simulink model "modlQuadcopter"  (R2024a)
settings: Solver=FixedStepAuto  StartTime=0.0  StopTime=CNFG_TEND  FixedStep=CNFG_TSTEP  RelTol=1e-3
undefined symbols (not defined in the file): BATT, CNST, DiscIntNeverNeededParam, MOTR, PROP, QUAD
libraries: vrlib x1, matrix_library x1
settings Model: Creator=anant  LastModifiedBy=anant

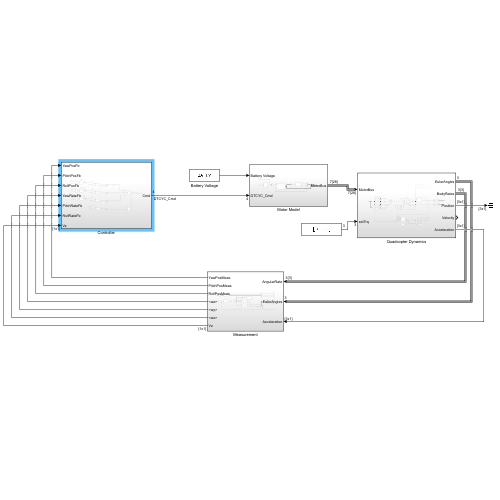
[thumbnail: Simulink's stored preview of the top-level diagram]
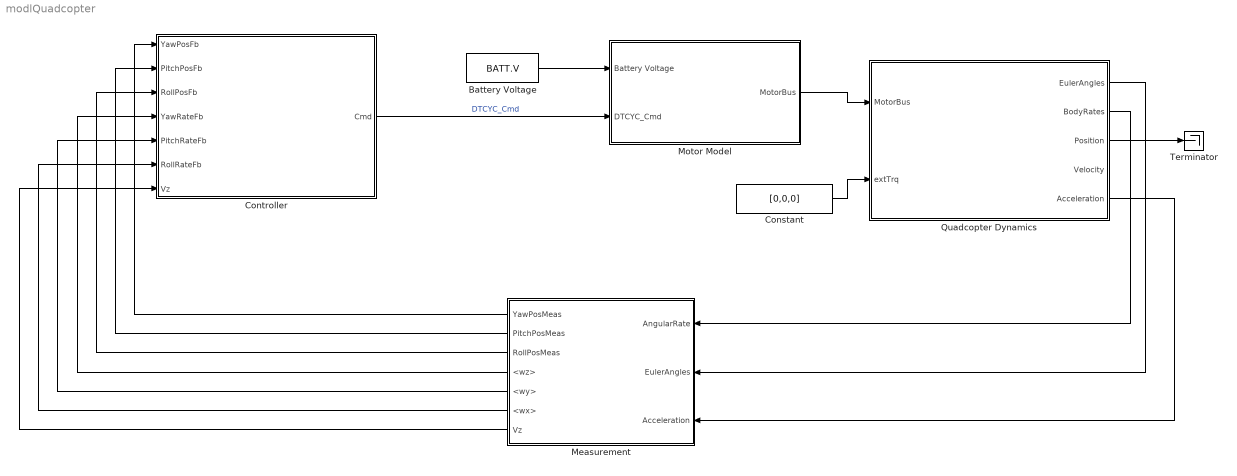
== system modlQuadcopter ==
  Battery Voltage : Constant  Value=BATT.V  SampleTime=0
  Constant : Constant  Value=[0,0,0]
  Controller : Subsystem
  Measurement : Subsystem
  Motor Model : Subsystem
  Quadcopter Dynamics : Subsystem
  Terminator : Terminator
  wires:
  Battery Voltage/1 -> Motor Model/1(Battery Voltage)
  Controller/1(Cmd) -> Motor Model/2(DTCYC_Cmd)  "DTCYC_Cmd"
  Motor Model/1(MotorBus) -> Quadcopter Dynamics/1(MotorBus)
  Quadcopter Dynamics/1(EulerAngles) -> Measurement/2(EulerAngles)
  Constant/1 -> Quadcopter Dynamics/2(extTrq)
  Quadcopter Dynamics/5(Acceleration) -> Measurement/3(Acceleration)
  Quadcopter Dynamics/2(BodyRates) -> Measurement/1(AngularRate)
  Measurement/1(YawPosMeas) -> Controller/1(YawPosFb)
  Measurement/2(PitchPosMeas) -> Controller/2(PitchPosFb)
  Measurement/3(RollPosMeas) -> Controller/3(RollPosFb)
  Measurement/4(<wz>) -> Controller/4(YawRateFb)
  Measurement/5(<wy>) -> Controller/5(PitchRateFb)
  Measurement/6(<wx>) -> Controller/6(RollRateFb)
  Measurement/7(Vz) -> Controller/7(Vz)
  Quadcopter Dynamics/3(Position) -> Terminator/1

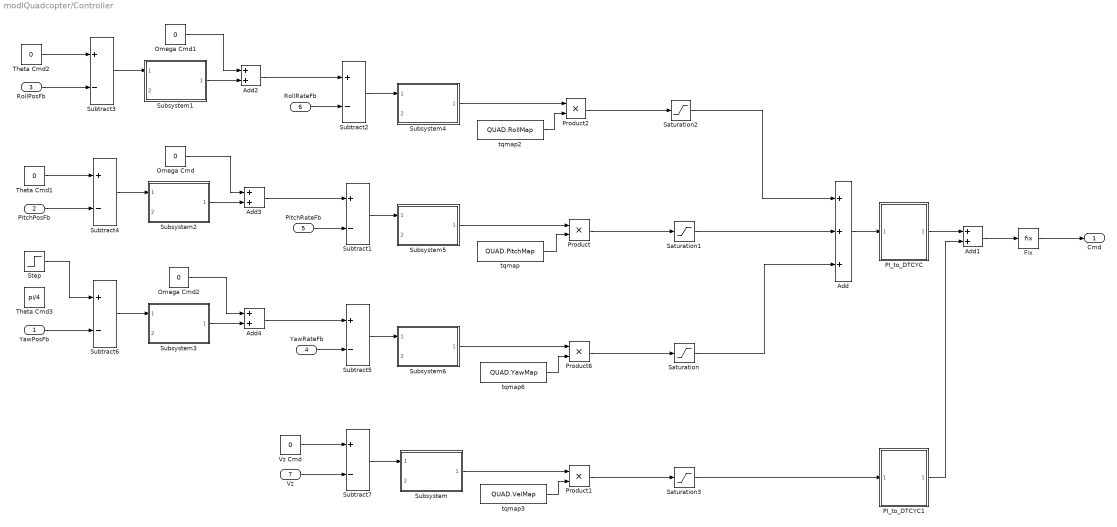
== system modlQuadcopter/Controller ==
  YawPosFb : Inport
  PitchPosFb : Inport  Port=2
  RollPosFb : Inport  Port=3
  YawRateFb : Inport  Port=4
  PitchRateFb : Inport  Port=5
  RollRateFb : Inport  Port=6
  Vz : Inport  Port=7
  Add : Sum  Inputs=+++
  Add{1..4} (4 alike) : Sum
  Fix : Rounding  Operator=fix
  Omega Cmd : Constant  Value=0
  Omega Cmd1 : Constant  Value=0
  Omega Cmd2 : Constant  Value=0
  PI_to_DTCYC : Subsystem  ReferencedSubsystem=subrMap  XL=-1  XU=1  YL=0  YU=500
  PI_to_DTCYC1 : Subsystem  ReferencedSubsystem=subrMap  XL=-1  XU=1  YL=1000  YU=2000
  Product{,1..2,6} (4 alike) : Product
  Saturation : Saturate  UpperLimit=0.2  LowerLimit=-0.2
  Saturation1 : Saturate  UpperLimit=0.4  LowerLimit=-0.4
  Saturation2 : Saturate  UpperLimit=0.4  LowerLimit=-0.4
  Saturation3 : Saturate  UpperLimit=1  LowerLimit=-1
  Step : Step  Time=0  After=0  SampleTime=0
  Subsystem : Subsystem  ReferencedSubsystem=subrPID  Kp=0.7  Ki=0.07  Kd=0  Ki_Sat=inf  TSTEP=CNTR.TSTEP
  Subsystem1 : Subsystem  ReferencedSubsystem=subrPID  Kp=20  Ki=0  Kd=0  Ki_Sat=inf  TSTEP=CNTR.TSTEP
  Subsystem2 : Subsystem  ReferencedSubsystem=subrPID  Kp=30  Ki=0  Kd=0  Ki_Sat=inf  TSTEP=CNTR.TSTEP
  Subsystem3 : Subsystem  ReferencedSubsystem=subrPID  Kp=5  Ki=0  Kd=0  Ki_Sat=inf  TSTEP=CNTR.TSTEP
  Subsystem4 : Subsystem  ReferencedSubsystem=subrPID  Kp=0.2  Ki=0  Kd=0  Ki_Sat=inf  TSTEP=CNTR.TSTEP
  Subsystem5 : Subsystem  ReferencedSubsystem=subrPID  Kp=0.2  Ki=0  Kd=0  Ki_Sat=inf  TSTEP=CNTR.TSTEP
  Subsystem6 : Subsystem  ReferencedSubsystem=subrPID  Kp=0.2  Ki=0  Kd=0  Ki_Sat=inf  TSTEP=CNTR.TSTEP
  Subtract{1..7} (7 alike) : Sum  Inputs=+-
  Theta Cmd1 : Constant  Value=0
  Theta Cmd2 : Constant  Value=0
  Theta Cmd3 : Constant  Value=pi/4
  Vz Cmd : Constant  Value=0
  tqmap : Constant  Value=QUAD.PitchMap
  tqmap2 : Constant  Value=QUAD.RollMap
  tqmap3 : Constant  Value=QUAD.VelMap
  tqmap6 : Constant  Value=QUAD.YawMap
  Cmd : Outport
  wires:
  Product6/1 -> Saturation/1
  Add2/1 -> Subtract2/1
  RollPosFb/1 -> Subtract3/2
  tqmap2/1 -> Product2/2
  tqmap6/1 -> Product6/2
  tqmap/1 -> Product/2
  RollRateFb/1 -> Subtract2/2
  Subtract2/1 -> Subsystem4/1
  Product/1 -> Saturation1/1
  PI_to_DTCYC/1 -> Add1/1
  Subtract1/1 -> Subsystem5/1
  Fix/1 -> Cmd/1
  PitchRateFb/1 -> Subtract1/2
  YawRateFb/1 -> Subtract5/2
  Product2/1 -> Saturation2/1
  Add/1 -> PI_to_DTCYC/1
  PI_to_DTCYC1/1 -> Add1/2
  Add1/1 -> Fix/1
  Add4/1 -> Subtract5/1
  Vz Cmd/1 -> Subtract7/1
  Vz/1 -> Subtract7/2
  Subtract7/1 -> Subsystem/1
  Subsystem/1 -> Product1/1
  tqmap3/1 -> Product1/2
  Product1/1 -> Saturation3/1
  Saturation3/1 -> PI_to_DTCYC1/1
  Subtract3/1 -> Subsystem1/1
  Omega Cmd1/1 -> Add2/1
  Theta Cmd2/1 -> Subtract3/1
  Subsystem1/1 -> Add2/2
  Omega Cmd/1 -> Add3/1
  Subsystem2/1 -> Add3/2
  Subtract4/1 -> Subsystem2/1
  PitchPosFb/1 -> Subtract4/2
  Theta Cmd1/1 -> Subtract4/1
  Add3/1 -> Subtract1/1
  Subsystem3/1 -> Add4/2
  YawPosFb/1 -> Subtract6/2
  Step/1 -> Subtract6/1
  Subsystem5/1 -> Product/1
  Subsystem6/1 -> Product6/1
  Subsystem4/1 -> Product2/1
  Omega Cmd2/1 -> Add4/1
  Saturation2/1 -> Add/1
  Saturation1/1 -> Add/2
  Saturation/1 -> Add/3
  Subtract5/1 -> Subsystem6/1
  Subtract6/1 -> Subsystem3/1

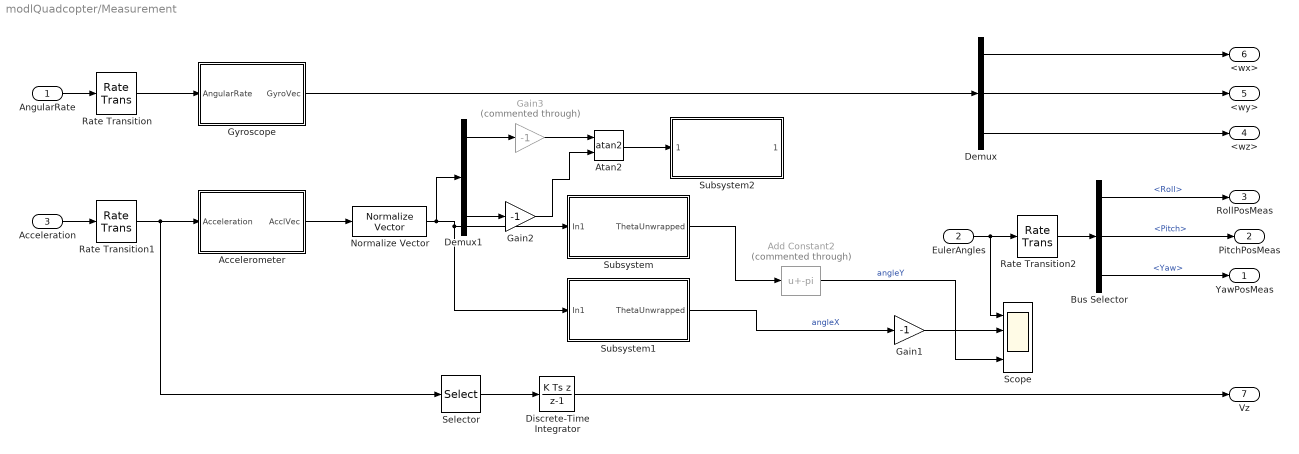
== system modlQuadcopter/Measurement ==
  AngularRate : Inport
  EulerAngles : Inport  Port=2
  Acceleration : Inport  Port=3
  Accelerometer : Subsystem
  Add Constant2 : Bias  Commented=through  Bias=-pi  SaturateOnIntegerOverflow=off
  Atan2 : Trigonometry  Operator=atan2
  Bus Selector : BusSelector  OutputSignals=Roll,Pitch,Yaw
  Demux : Demux  Outputs=3
  Demux1 : Demux  Outputs=3
  Discrete-Time Integrator : DiscreteIntegrator  IntegratorMethod=Integration: Backward Euler  SampleTime=-1  ICPrevOutput=DiscIntNeverNeededParam  ICPrevScaledInput=DiscIntNeverNeededParam
  Gain1 : Gain  Gain=-1
  Gain2 : Gain  Gain=-1
  Gain3 : Gain  Commented=through  Gain=-1
  Gyroscope : Subsystem
  Normalize Vector : vrlib/Utilities/Normalize Vector  maxzero=0
  Rate Transition : RateTransition  OutPortSampleTime=CNTR.TSTEP
  Rate Transition1 : RateTransition  OutPortSampleTime=CNTR.TSTEP
  Rate Transition2 : RateTransition  OutPortSampleTime=CNTR.TSTEP
  Scope : Scope  NumInputPorts=4
  Selector : Selector  InputPortWidth=3  IndexOptions=Index vector (dialog)  Indices=[3]  OutputSizes=1
  Subsystem : Subsystem
  Subsystem1 : Subsystem
  Subsystem2 : Subsystem  ReferencedSubsystem=subrUnwrap
  YawPosMeas : Outport
  PitchPosMeas : Outport  Port=2
  RollPosMeas : Outport  Port=3
  <wz> : Outport  Port=4
  <wy> : Outport  Port=5
  <wx> : Outport  Port=6
  Vz : Outport  Port=7
  wires:
  AngularRate/1 -> Rate Transition/1
  Gyroscope/1(GyroVec) -> Demux/1
  Demux/1 -> <wx>/1
  Demux/2 -> <wy>/1
  Demux/3 -> <wz>/1
  EulerAngles/1 -> Scope/1, Rate Transition2/1
  Bus Selector/1 -> RollPosMeas/1  "<Roll>"
  Bus Selector/2 -> PitchPosMeas/1  "<Pitch>"
  Bus Selector/3 -> YawPosMeas/1  "<Yaw>"
  Acceleration/1 -> Rate Transition1/1
  Accelerometer/1(AcclVec) -> Normalize Vector/1
  Rate Transition/1 -> Gyroscope/1(AngularRate)
  Rate Transition1/1 -> Selector/1, Accelerometer/1(Acceleration)
  Rate Transition2/1 -> Bus Selector/1
  Discrete-Time Integrator/1 -> Vz/1
  Selector/1 -> Discrete-Time Integrator/1
  Atan2/1 -> Subsystem2/1
  Subsystem1/1(ThetaUnwrapped) -> Gain1/1  "angleX"
  Add Constant2/1 -> Scope/4  "angleY"
  Gain1/1 -> Scope/2
  Normalize Vector/1 -> Demux1/1, Subsystem1/1(In1), Subsystem/1(In1)
  Subsystem/1(ThetaUnwrapped) -> Add Constant2/1
  Gain3/1 -> Atan2/1
  Gain2/1 -> Atan2/2
  Demux1/3 -> Gain2/1
  Demux1/1 -> Gain3/1

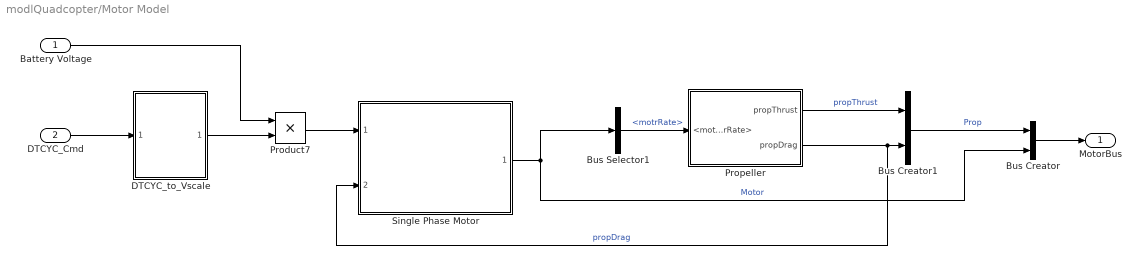
== system modlQuadcopter/Motor Model ==
  Battery Voltage : Inport
  DTCYC_Cmd : Inport  Port=2
  Bus Creator : BusCreator  Inputs=2
  Bus Creator1 : BusCreator  Inputs=2
  Bus Selector1 : BusSelector  OutputSignals=motrRate
  DTCYC_to_Vscale : Subsystem  ReferencedSubsystem=subrMap  XL=1000  XU=2000  YL=0  YU=1
  Product7 : Product
  Propeller : Subsystem
  Single Phase Motor : Subsystem  ReferencedSubsystem=subrSinglePhaseMotor  RL=MOTR.RL  LL=MOTR.LL  KB=MOTR.KB  KT=MOTR.KT  J=MOTR.J  B=MOTR.B  D=MOTR.D
  MotorBus : Outport
  wires:
  DTCYC_to_Vscale/1 -> Product7/2
  Propeller/2(propDrag) -> Single Phase Motor/2, Bus Creator1/2  "propDrag"
  Bus Selector1/1 -> Propeller/1(<motrRate>)  "<motrRate>"
  Propeller/1(propThrust) -> Bus Creator1/1  "propThrust"
  Single Phase Motor/1 -> Bus Creator/2, Bus Selector1/1  "Motor"
  Product7/1 -> Single Phase Motor/1
  Battery Voltage/1 -> Product7/1
  DTCYC_Cmd/1 -> DTCYC_to_Vscale/1
  Bus Creator/1 -> MotorBus/1
  Bus Creator1/1 -> Bus Creator/1  "Prop"

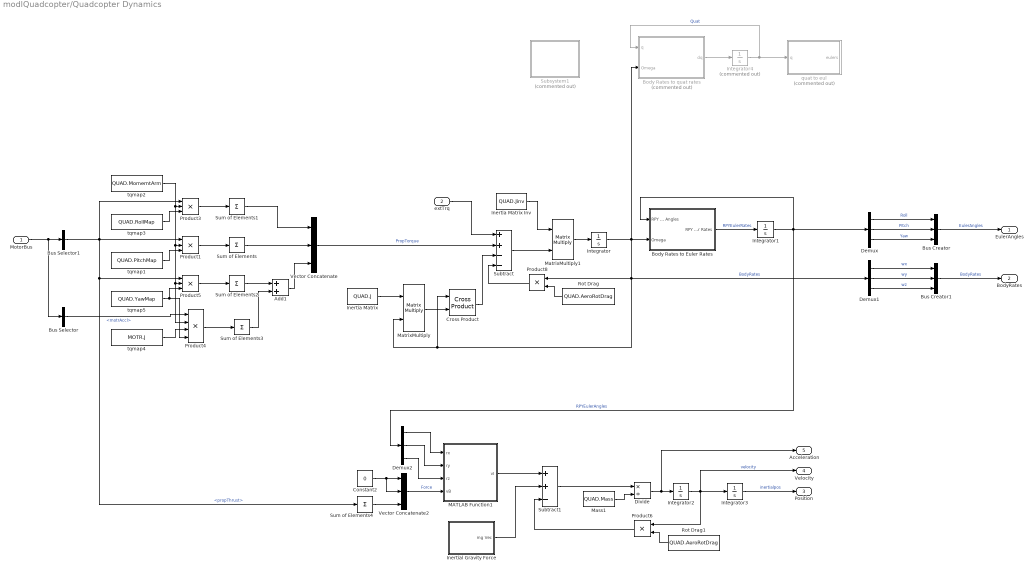
== system modlQuadcopter/Quadcopter Dynamics ==
  MotorBus : Inport
  extTrq : Inport  Port=2
  Add1 : Sum
  Body Rates to Euler Rates : Subsystem
  Body Rates to quat rates : Subsystem  Commented=on
  Bus Creator : BusCreator  Inputs=3
  Bus Creator1 : BusCreator  Inputs=3
  Bus Selector : BusSelector  OutputSignals=Motor.motrAccl
  Bus Selector1 : BusSelector  OutputSignals=Prop.propThrust
  Constant2 : Constant  Value=0
  Cross Product : matrix_library/Cross Product
  Demux : Demux  Outputs=3
  Demux1 : Demux  Outputs=3
  Demux2 : Demux  Outputs=3
  Divide : Product  Inputs=*/
  Inertia Matrix : Constant  Value=QUAD.J
  Inertia Matrix Inv : Constant  Value=QUAD.Jinv
  Inertial Gravity Force : Subsystem
  Integrator : Integrator
  Integrator1 : Integrator  InitialCondition=[0,0,0]
  Integrator2 : Integrator
  Integrator3 : Integrator
  Integrator4 : Integrator  Commented=on  InitialCondition=[1,0,0,0]
  MATLAB Function1 : MATLAB Function  TreatAsAtomicUnit=on
  Mass1 : Constant  Value=QUAD.Mass
  MatrixMultiply : Product  Multiplication=Matrix(*)
  MatrixMultiply1 : Product  Multiplication=Matrix(*)
  Product1 : Product  Inputs=3
  Product3 : Product  Inputs=3
  Product4 : Product  Inputs=4
  Product5 : Product  Inputs=3
  Product6 : Product
  Product8 : Product
  Rot Drag : Constant  Value=QUAD.AeroRotDrag
  Rot Drag1 : Constant  Value=QUAD.AeroRotDrag
  Subsystem1 : Subsystem  Commented=on
  Subtract : Sum  Inputs=++--
  Subtract1 : Sum  Inputs=++-
  Sum of Elements{,1..4} (5 alike) : Sum  Inputs=+
  Vector Concatenate : Concatenate  NumInputs=3
  Vector Concatenate2 : Concatenate  NumInputs=3
  quat to eul : Subsystem  Commented=on
  tqmap1 : Constant  Value=QUAD.PitchMap
  tqmap2 : Constant  Value=QUAD.MomemtArm
  tqmap3 : Constant  Value=QUAD.RollMap
  tqmap4 : Constant  Value=MOTR.J
  tqmap5 : Constant  Value=QUAD.YawMap
  EulerAngles : Outport
  BodyRates : Outport  Port=2
  Position : Outport  Port=3
  Velocity : Outport  Port=4
  Acceleration : Outport  Port=5
  wires:
  Bus Selector1/1 -> Sum of Elements4/1, Product5/1, Product3/1, Product1/1  "<propThrust>"
  Product5/1 -> Sum of Elements2/1
  MatrixMultiply/1 -> Cross Product/2
  tqmap3/1 -> Product3/3
  MotorBus/1 -> Bus Selector/1, Bus Selector1/1
  Integrator/1 -> Body Rates to quat rates/2(Omega), Cross Product/1, MatrixMultiply/2, Demux1/1, Product8/1, Body Rates to Euler Rates/2(Omega)  "BodyRates"
  tqmap5/1 -> Product4/4, Product5/3
  Product3/1 -> Sum of Elements1/1
  Inertia Matrix Inv/1 -> MatrixMultiply1/1
  Rot Drag/1 -> Product8/2
  Product8/1 -> Subtract/4
  Inertia Matrix/1 -> MatrixMultiply/1
  Sum of Elements3/1 -> Add1/2
  tqmap4/1 -> Product4/3
  Product4/1 -> Sum of Elements3/1
  tqmap1/1 -> Product1/3
  Product1/1 -> Sum of Elements/1
  Vector Concatenate/1 -> Subtract/2  "PropTorque"
  MatrixMultiply1/1 -> Integrator/1
  Sum of Elements/1 -> Vector Concatenate/2
  Add1/1 -> Vector Concatenate/3
  Cross Product/1 -> Subtract/3
  Sum of Elements1/1 -> Vector Concatenate/1
  Sum of Elements2/1 -> Add1/1
  Body Rates to Euler Rates/1(RPY Euler Rates) -> Integrator1/1  "RPYEulerRates"
  Bus Selector/1 -> Product4/1  "<motrAccl>"
  Integrator1/1 -> Body Rates to Euler Rates/1(RPY Euler Angles), Demux/1, Demux2/1  "RPYEulerAngles"
  Constant2/1 -> Vector Concatenate2/2, Vector Concatenate2/1
  Sum of Elements4/1 -> Vector Concatenate2/3
  Vector Concatenate2/1 -> MATLAB Function1/4(vB)  "Force"
  Demux2/3 -> MATLAB Function1/3(rz)
  Demux2/2 -> MATLAB Function1/2(ry)
  Demux2/1 -> MATLAB Function1/1(rx)
  MATLAB Function1/1(vI) -> Subtract1/1
  Rot Drag1/1 -> Product6/2
  Subtract1/1 -> Divide/1
  Integrator2/1 -> Product6/1, Velocity/1, Integrator3/1  "velocity"
  Product6/1 -> Subtract1/3
  Divide/1 -> Acceleration/1, Integrator2/1
  Mass1/1 -> Divide/2
  Integrator3/1 -> Position/1  "inertialpos"
  tqmap2/1 -> Product4/2, Product5/2, Product1/2, Product3/2
  extTrq/1 -> Subtract/1
  Inertial Gravity Force/1(mg Vec) -> Subtract1/2
  Body Rates to quat rates/1(dq) -> Integrator4/1
  Integrator4/1 -> quat to eul/1(q), Body Rates to quat rates/1(q)  "Quat"
  Demux/1 -> Bus Creator/1  "Roll"
  Demux/2 -> Bus Creator/2  "Pitch"
  Demux/3 -> Bus Creator/3  "Yaw"
  Bus Creator/1 -> EulerAngles/1  "EulerAngles"
  Demux1/3 -> Bus Creator1/3  "wz"
  Demux1/1 -> Bus Creator1/1  "wx"
  Demux1/2 -> Bus Creator1/2  "wy"
  Bus Creator1/1 -> BodyRates/1  "BodyRates"
  Subtract/1 -> MatrixMultiply1/2

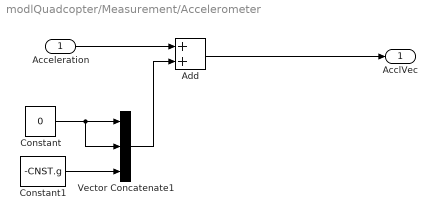
== system modlQuadcopter/Measurement/Accelerometer ==
  Acceleration : Inport
  Add : Sum
  Constant : Constant  Value=0
  Constant1 : Constant  Value=-CNST.g
  Vector Concatenate1 : Concatenate  NumInputs=3
  AcclVec : Outport
  wires:
  Vector Concatenate1/1 -> Add/2
  Acceleration/1 -> Add/1
  Constant/1 -> Vector Concatenate1/2, Vector Concatenate1/1
  Constant1/1 -> Vector Concatenate1/3
  Add/1 -> AcclVec/1

== system modlQuadcopter/Measurement/Gyroscope ==
  AngularRate : Inport
  GyroVec : Outport
  wires:
  AngularRate/1 -> GyroVec/1

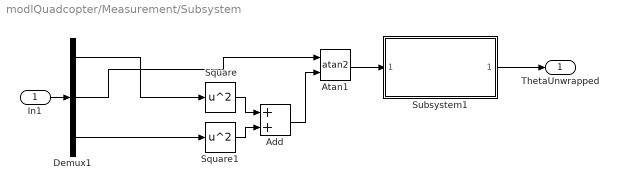
== system modlQuadcopter/Measurement/Subsystem ==
  In1 : Inport
  Add : Sum
  Atan1 : Trigonometry  Operator=atan2
  Demux1 : Demux  Outputs=3
  Square : Math  Operator=square
  Square1 : Math  Operator=square
  Subsystem1 : Subsystem  ReferencedSubsystem=subrUnwrap
  ThetaUnwrapped : Outport
  wires:
  Demux1/2 -> Atan1/1
  Square1/1 -> Add/2
  Atan1/1 -> Subsystem1/1
  Square/1 -> Add/1
  Add/1 -> Atan1/2
  Subsystem1/1 -> ThetaUnwrapped/1
  In1/1 -> Demux1/1
  Demux1/1 -> Square/1
  Demux1/3 -> Square1/1

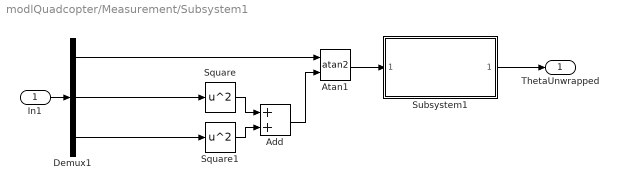
== system modlQuadcopter/Measurement/Subsystem1 ==
  In1 : Inport
  Add : Sum
  Atan1 : Trigonometry  Operator=atan2
  Demux1 : Demux  Outputs=3
  Square : Math  Operator=square
  Square1 : Math  Operator=square
  Subsystem1 : Subsystem  ReferencedSubsystem=subrUnwrap
  ThetaUnwrapped : Outport
  wires:
  Demux1/3 -> Square1/1
  In1/1 -> Demux1/1
  Subsystem1/1 -> ThetaUnwrapped/1
  Add/1 -> Atan1/2
  Square/1 -> Add/1
  Atan1/1 -> Subsystem1/1
  Square1/1 -> Add/2
  Demux1/1 -> Atan1/1
  Demux1/2 -> Square/1

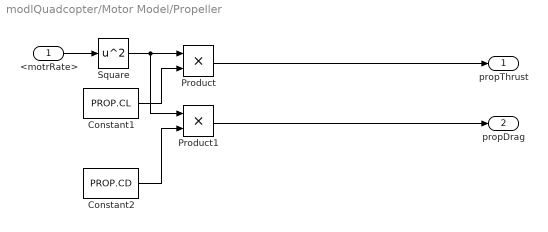
== system modlQuadcopter/Motor Model/Propeller ==
  <motrRate> : Inport
  Constant1 : Constant  Value=PROP.CL
  Constant2 : Constant  Value=PROP.CD
  Product : Product
  Product1 : Product
  Square : Math  Operator=square
  propThrust : Outport
  propDrag : Outport  Port=2
  wires:
  Square/1 -> Product/1, Product1/1
  Constant1/1 -> Product/2
  Product/1 -> propThrust/1
  <motrRate>/1 -> Square/1
  Constant2/1 -> Product1/2
  Product1/1 -> propDrag/1

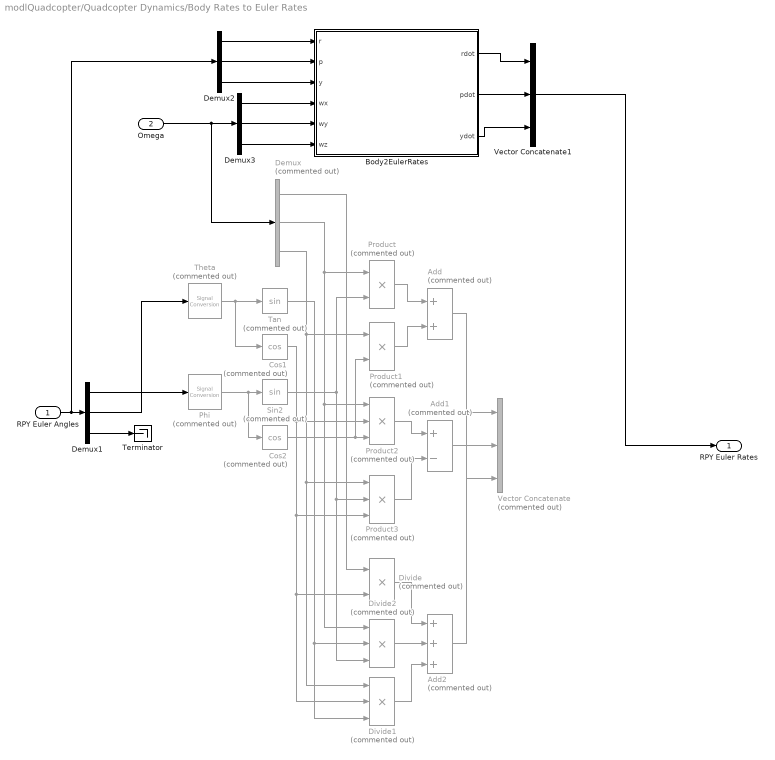
== system modlQuadcopter/Quadcopter Dynamics/Body Rates to Euler Rates ==
  RPY Euler Angles : Inport
  Omega : Inport  Port=2
  Add : Sum  Commented=on
  Add1 : Sum  Commented=on  Inputs=+-
  Add2 : Sum  Commented=on  Inputs=+++
  Body2EulerRates : MATLAB Function  TreatAsAtomicUnit=on
  Cos1 : Trigonometry  Commented=on  Operator=cos
  Cos2 : Trigonometry  Commented=on  Operator=cos
  Demux : Demux  Commented=on  Outputs=3
  Demux1 : Demux  Outputs=3
  Demux2 : Demux  Outputs=3
  Demux3 : Demux  Outputs=3
  Divide : Product  Commented=on  Inputs=**
  Divide1 : Product  Commented=on  Inputs=***
  Divide2 : Product  Commented=on  Inputs=***
  Phi : SignalConversion  Commented=on  OverrideOpt=off
  Product : Product  Commented=on
  Product1 : Product  Commented=on
  Product2 : Product  Commented=on  Inputs=3
  Product3 : Product  Commented=on  Inputs=3
  Sin2 : Trigonometry  Commented=on
  Tan : Trigonometry  Commented=on
  Terminator : Terminator
  Theta : SignalConversion  Commented=on  OverrideOpt=off
  Vector Concatenate : Concatenate  Commented=on  NumInputs=3
  Vector Concatenate1 : Concatenate  NumInputs=3
  RPY Euler Rates : Outport
  wires:
  Demux1/2 -> Theta/1
  Omega/1 -> Demux/1, Demux3/1
  Demux1/1 -> Phi/1
  Phi/1 -> Sin2/1, Cos2/1
  Theta/1 -> Tan/1, Cos1/1
  Add/1 -> Vector Concatenate/3
  Add1/1 -> Vector Concatenate/2
  Add2/1 -> Vector Concatenate/1
  Sin2/1 -> Divide2/3, Product3/2, Product/2
  Cos2/1 -> Product1/2, Product2/3
  Demux/2 -> Divide2/1, Product2/1, Product/1
  Demux/3 -> Divide1/1, Product3/1, Product1/1
  Product/1 -> Add/1
  Product1/1 -> Add/2
  Cos1/1 -> Divide1/2, Divide/2, Product3/3, Product2/2
  Demux/1 -> Divide/1
  Divide2/1 -> Add2/2
  Divide/1 -> Add2/1
  Divide1/1 -> Add2/3
  Tan/1 -> Divide1/3, Divide2/2
  Product2/1 -> Add1/1
  Product3/1 -> Add1/2
  Demux1/3 -> Terminator/1
  RPY Euler Angles/1 -> Demux2/1, Demux1/1
  Body2EulerRates/2(pdot) -> Vector Concatenate1/2
  Body2EulerRates/1(rdot) -> Vector Concatenate1/1
  Body2EulerRates/3(ydot) -> Vector Concatenate1/3
  Demux3/1 -> Body2EulerRates/4(wx)
  Demux3/2 -> Body2EulerRates/5(wy)
  Demux3/3 -> Body2EulerRates/6(wz)
  Demux2/1 -> Body2EulerRates/1(r)
  Demux2/2 -> Body2EulerRates/2(p)
  Demux2/3 -> Body2EulerRates/3(y)
  Vector Concatenate1/1 -> RPY Euler Rates/1

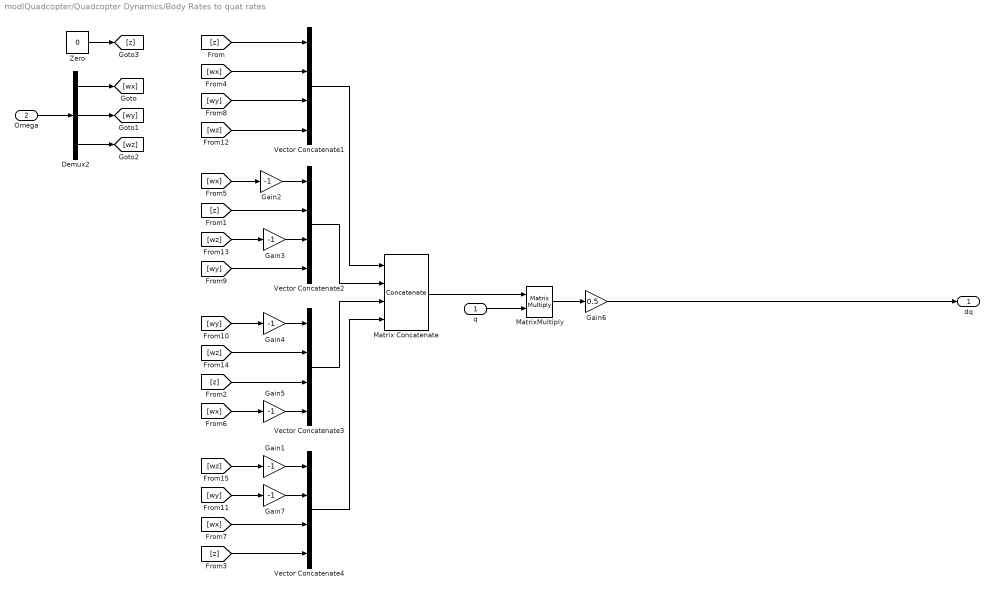
== system modlQuadcopter/Quadcopter Dynamics/Body Rates to quat rates ==
  q : Inport
  Omega : Inport  Port=2
  Demux2 : Demux  Outputs=3
  Gain{1..5,7} (6 alike) : Gain  Gain=-1
  Gain6 : Gain  Gain=0.5
  Matrix Concatenate : Concatenate  NumInputs=4  Mode=Multidimensional array  ConcatenateDimension=2
  MatrixMultiply : Product  Multiplication=Matrix(*)
  Vector Concatenate{1..4} (4 alike) : Concatenate  NumInputs=4
  Zero : Constant  Value=0  OutDataTypeStr=Inherit: Inherit via back propagation
  dq : Outport
  wires:
  Omega/1 -> Demux2/1
  Demux2/1 -> [wx]
  Demux2/2 -> [wy]
  Demux2/3 -> [wz]
  Zero/1 -> [z]
  [z] -> Vector Concatenate2/2
  [z] -> Vector Concatenate3/3
  [z] -> Vector Concatenate4/4
  [wz] -> Vector Concatenate1/4
  [wz] -> Gain3/1
  Gain3/1 -> Vector Concatenate2/3
  [wz] -> Vector Concatenate3/2
  [wz] -> Gain1/1
  [wy] -> Vector Concatenate1/3
  [wy] -> Vector Concatenate2/4
  [wy] -> Gain4/1
  Gain4/1 -> Vector Concatenate3/1
  [wy] -> Gain7/1
  [z] -> Vector Concatenate1/1
  [wx] -> Vector Concatenate1/2
  [wx] -> Gain2/1
  [wx] -> Gain5/1
  Gain5/1 -> Vector Concatenate3/4
  [wx] -> Vector Concatenate4/3
  Vector Concatenate1/1 -> Matrix Concatenate/1
  Vector Concatenate2/1 -> Matrix Concatenate/2
  Vector Concatenate3/1 -> Matrix Concatenate/3
  Vector Concatenate4/1 -> Matrix Concatenate/4
  Matrix Concatenate/1 -> MatrixMultiply/1
  q/1 -> MatrixMultiply/2
  MatrixMultiply/1 -> Gain6/1
  Gain6/1 -> dq/1
  Gain2/1 -> Vector Concatenate2/1
  Gain1/1 -> Vector Concatenate4/1
  Gain7/1 -> Vector Concatenate4/2

== system modlQuadcopter/Quadcopter Dynamics/Inertial Gravity Force ==
  Constant : Constant  Value=0
  Constant1 : Constant  Value=-CNST.g
  Mass : Constant  Value=QUAD.Mass
  Product2 : Product
  Vector Concatenate1 : Concatenate  NumInputs=3
  mg Vec : Outport
  wires:
  Constant1/1 -> Vector Concatenate1/3
  Constant/1 -> Vector Concatenate1/2, Vector Concatenate1/1
  Vector Concatenate1/1 -> Product2/2  "gravity"
  Product2/1 -> mg Vec/1
  Mass/1 -> Product2/1

== system modlQuadcopter/Quadcopter Dynamics/Subsystem1 ==
  MATLAB Function : MATLAB Function  Commented=on  TreatAsAtomicUnit=on

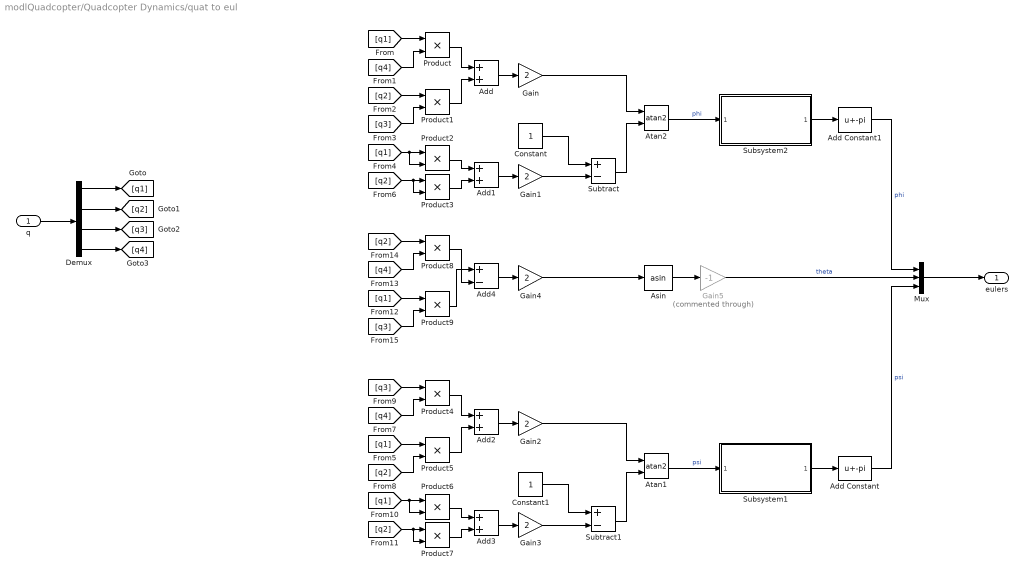
== system modlQuadcopter/Quadcopter Dynamics/quat to eul ==
  q : Inport
  Add{,1..3} (4 alike) : Sum
  Add Constant : Bias  Bias=-pi  SaturateOnIntegerOverflow=off
  Add Constant1 : Bias  Bias=-pi  SaturateOnIntegerOverflow=off
  Add4 : Sum  Inputs=+-
  Asin : Trigonometry  Operator=asin
  Atan1 : Trigonometry  Operator=atan2
  Atan2 : Trigonometry  Operator=atan2
  Constant : Constant
  Constant1 : Constant
  Demux : Demux
  Gain{,1..4} (5 alike) : Gain  Gain=2
  Gain5 : Gain  Commented=through  Gain=-1
  Mux : Mux  Inputs=3
  Product{,1..9} (10 alike) : Product
  Subsystem1 : Subsystem  ReferencedSubsystem=subrUnwrap
  Subsystem2 : Subsystem  ReferencedSubsystem=subrUnwrap
  Subtract : Sum  Inputs=+-
  Subtract1 : Sum  Inputs=+-
  eulers : Outport
  wires:
  q/1 -> Demux/1
  Demux/1 -> [q1]
  Demux/2 -> [q2]
  Demux/3 -> [q3]
  Demux/4 -> [q4]
  Product/1 -> Add/1
  Product1/1 -> Add/2
  [q1] -> Product/1
  [q4] -> Product/2
  [q2] -> Product1/1
  [q3] -> Product1/2
  Add/1 -> Gain/1
  Gain/1 -> Atan2/1
  [q1] -> Product2/2, Product2/1
  [q2] -> Product3/2, Product3/1
  Product2/1 -> Add1/1
  Product3/1 -> Add1/2
  Add1/1 -> Gain1/1
  Constant/1 -> Subtract/1
  Gain1/1 -> Subtract/2
  Subtract/1 -> Atan2/2
  Subtract1/1 -> Atan1/2
  Add3/1 -> Gain3/1
  [q2] -> Product7/2, Product7/1
  Product7/1 -> Add3/2
  [q3] -> Product4/1
  [q1] -> Product6/2, Product6/1
  Product6/1 -> Add3/1
  Add2/1 -> Gain2/1
  Constant1/1 -> Subtract1/1
  [q4] -> Product4/2
  [q2] -> Product5/2
  Product4/1 -> Add2/1
  Product5/1 -> Add2/2
  Gain3/1 -> Subtract1/2
  [q1] -> Product5/1
  Gain2/1 -> Atan1/1
  Atan1/1 -> Subsystem1/1  "psi"
  [q2] -> Product8/1
  [q4] -> Product8/2
  [q3] -> Product9/2
  Product8/1 -> Add4/2
  Product9/1 -> Add4/1
  [q1] -> Product9/1
  Gain4/1 -> Asin/1
  Add4/1 -> Gain4/1
  Asin/1 -> Gain5/1
  Atan2/1 -> Subsystem2/1  "phi"
  Subsystem2/1 -> Add Constant1/1
  Subsystem1/1 -> Add Constant/1
  Gain5/1 -> Mux/2  "theta"
  Add Constant/1 -> Mux/3  "psi"
  Add Constant1/1 -> Mux/1  "phi"
  Mux/1 -> eulers/1

== matlab function modlQuadcopter/Quadcopter Dynamics/MATLAB Function1 ==
  data: rx input; vI output; ry input; rz input; vB input
function vI = RotateB2I(rx,ry,rz,vB)
    C = RotXB2I(rx) * RotYB2I(ry) * RotZB2I(rz);
    vI = (vB'*C)';
end

function [mat] = RotZB2I(t)
    mat = [cos(t), -sin(t), 0;...
        sin(t), cos(t), 0;...
        0,0,1];
end

function [mat] = RotYB2I(t)
    mat = [cos(t),0, sin(t);...
        0,1,0;...
        -sin(t), 0, cos(t)];
end

function [mat] = RotXB2I(t)
    mat = [1,0,0;...
        0,cos(t), -sin(t);...
        0,sin(t), cos(t)];
end

== matlab function modlQuadcopter/Quadcopter Dynamics/Subsystem1/MATLAB Function ==
  data: rx input; vB output; ry input; rz input; vI input
function vB = RotateI2B(rx,ry,rz,vI)
    C = RotZI2B(rz) * RotYI2B(ry) * RotXI2B(rx);
    vB = (vI'*C)';

end

function [mat] = RotZI2B(t)
% I to B
    mat = [cos(t), sin(t), 0;...
        -sin(t), cos(t), 0;...
        0,0,1];
end

function [mat] = RotYI2B(t)
% I to B
    mat = [cos(t),0, -sin(t);...
        0,1,0;...
        sin(t), 0, cos(t)];
end

function [mat] = RotXI2B(t)
% I to B
    mat = [1,0,0;...
        0,cos(t), sin(t);...
        0,-sin(t), cos(t)];
end

== matlab function modlQuadcopter/Quadcopter Dynamics/Body Rates to Euler Rates/Body2EulerRates ==
  data: r input; rdot output; p input; y input; wx input; wy input; wz input; pdot output; ydot output
function [rdot,pdot,ydot] = fcn(r,p,y,wx,wy,wz)
   w = [wx,wy,wz]';
   C = [1,  sin(y)*tan(p),  cos(y)*tan(p);...
       0,   cos(y),         -sin(y);...
       0, sin(y)/cos(p),    cos(y)/cos(p)];
   out = C*w;
   rdot = out(1);
   pdot = out(2);
   ydot = out(3);

end
